simulink model "variableRelactanceSM"  (R2023a)
settings: Solver=VariableStepAuto  StartTime=0.0  StopTime=10.0  RelTol=1e-3
libraries: spsIdealSwitchLib x3, spsDCVoltageSourceLib x1, spsStepperMotorLib x1, sps_lib x1
settings Model: Creator=Hp  LastModifiedBy=Hp

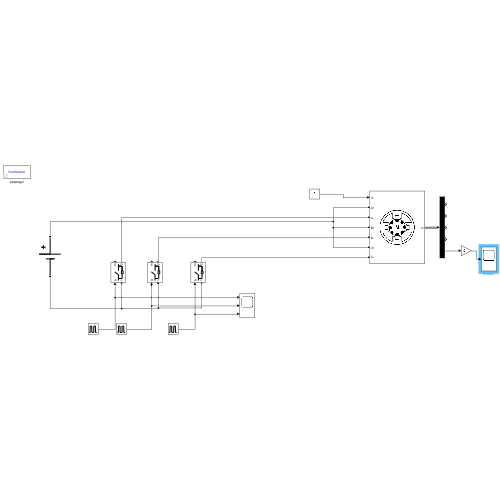
[thumbnail: Simulink's stored preview of the top-level diagram]
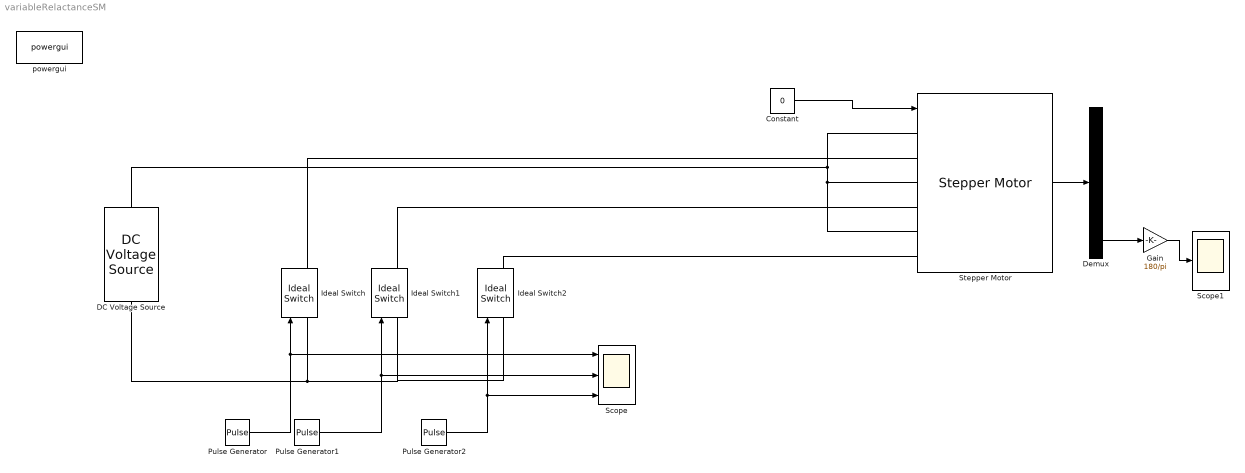
== system variableRelactanceSM ==
  Constant : Constant  Value=0
  DC Voltage Source : spsDCVoltageSourceLib/DC Voltage Source  Amplitude=25  Measurements=None
  Demux : Demux  Outputs=5
  Gain : Gain  Gain=180/pi
  Ideal Switch : spsIdealSwitchLib/Ideal Switch  Ron=0.001  Lon=0  IC=0  Rs=1e5  Cs=inf  Measurements=on
  Ideal Switch1 : spsIdealSwitchLib/Ideal Switch  Ron=0.001  Lon=0  IC=0  Rs=1e5  Cs=inf  Measurements=on
  Ideal Switch2 : spsIdealSwitchLib/Ideal Switch  Ron=0.001  Lon=0  IC=0  Rs=1e5  Cs=inf  Measurements=on
  Pulse Generator : DiscretePulseGenerator  PulseType=Time based  Period=6  PulseWidth=50
  Pulse Generator1 : DiscretePulseGenerator  PulseType=Time based  Period=6  PulseWidth=50  PhaseDelay=2
  Pulse Generator2 : DiscretePulseGenerator  PulseType=Time based  Period=6  PulseWidth=50  PhaseDelay=-2
  Scope : Scope  NumInputPorts=3
  Scope1 : Scope
  Stepper Motor : spsStepperMotorLib/Stepper Motor  MotorType=Variable reluctance  NumberOfPhases_1=2  NumberOfPhases_2=3  PresetModel_1=<empty>  PresetModel_2=<empty>  L=10e-3  Lmax=10e-3  Lmin=2e-3  R=1.2  Step_angle=30  Psim=0.04  Tdm=0.02  J=1e-4/5  B=1e-3  w0=0  pos0=0  TsPowergui=0  TsBlock=-1
      settings: LibrarySourceBlock=sps_lib/Electrical Machines/Stepper Motor
  powergui : sps_lib/powergui  Priority=1  SimulationMode=Continuous  SampleTime=50e-6  frequency=60  Iterations=50  frequencyindice=0  Pbase=100e6  ErrMax=1e-4  UnitsV=kV  UnitsW=MW  buscounter=0  FunctionMessages=off  echomessages=off  EnableUseOfTLC=off  CurrentSourceSwitches=off  DisableSnubberDevices=off  DisableRonSwitches=off  DisableVfSwitches=off  DisplayEquations=off  AutomaticDiscreteSolvers=off  SolverType=Tustin/Backward Euler (TBE)  Interpol=off  ExternalGateDelay=off  methode=off  Ts=100  x0status=blocks  SPID=on  SwTol=0  HookPort=off  NonlinearTolerance=1e-4  nMaxIteration=100  ContinueOnMaxIteration=off  RestoreLinks=warning  ResistiveCurrentMeasurement=off  Frange=[0:2:500]  Ylog=off  Xlog=on  ShowGrid=off  save=off  variable=ZData  structure=0  ZoomFFT=off  StartTime=0.0  cycles=1  DisplayStyle=1  fundamental=60  FreqAxis=off  MaxFrequency=1000  frequencyindicesteady=1  RmsSteady=1  display=off
  wires:
  Constant/1 -> Stepper Motor/1
  Pulse Generator/1 -> Scope/1, Ideal Switch/1
  Stepper Motor/1 -> Demux/1
  Demux/5 -> Gain/1
  Gain/1 -> Scope1/1
  Pulse Generator1/1 -> Scope/2, Ideal Switch1/1
  Pulse Generator2/1 -> Scope/3, Ideal Switch2/1
  connections:
  Stepper Motor/LConn1 -- DC Voltage Source/RConn1 -- Stepper Motor/LConn5 -- Stepper Motor/LConn3
  Ideal Switch/RConn1 -- Stepper Motor/LConn2
  Ideal Switch1/RConn1 -- Stepper Motor/LConn4
  Ideal Switch2/RConn1 -- Stepper Motor/LConn6
  DC Voltage Source/LConn1 -- Ideal Switch2/LConn1 -- Ideal Switch1/LConn1 -- Ideal Switch/LConn1
